simulink model "zoh"  (R2024b)
settings: Solver=VariableStepAuto  StartTime=0.0  StopTime=10.0  RelTol=1e-3
undefined symbols (not defined in the file or in its folder): drv, gbox, mld, mot, PID, rads2rpm, sens, sIn, specs
libraries: simulink_extras x6
settings Model: Creator=Nihal  LastModifiedBy=Nihal

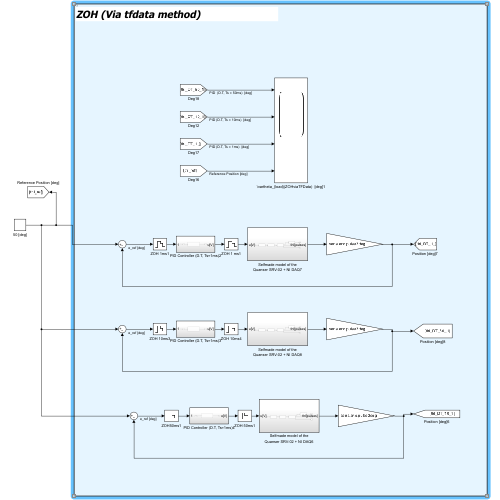
[thumbnail: Simulink's stored preview of the top-level diagram]
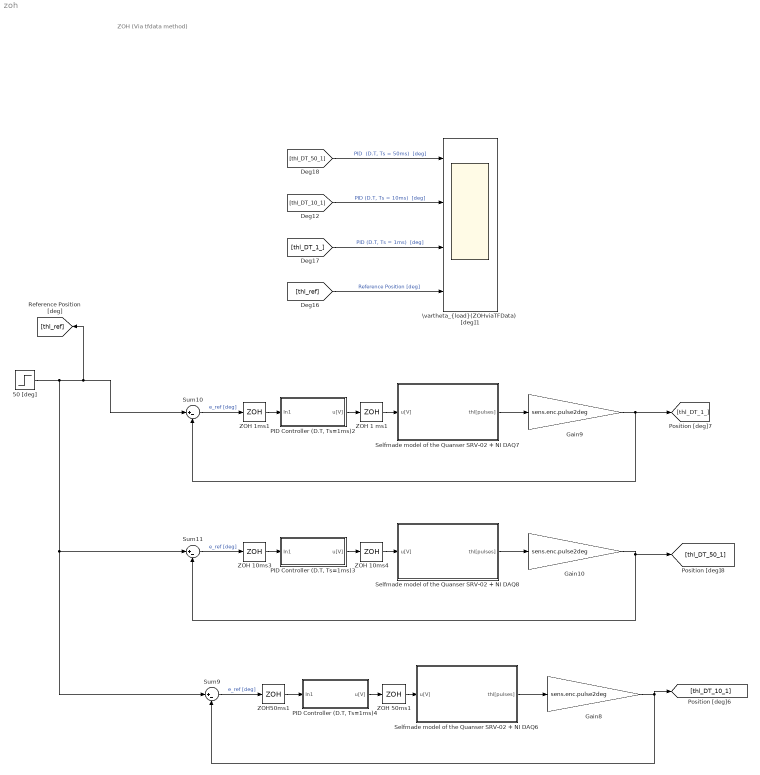
== system zoh ==
  note: ZOH (Via tfdata method)
  50 [deg] : Step  Time=0  After=sIn.position(1)  SampleTime=0
  Gain10 : Gain  Gain=sens.enc.pulse2deg
  Gain8 : Gain  Gain=sens.enc.pulse2deg
  Gain9 : Gain  Gain=sens.enc.pulse2deg
  "PID Controller (D.T, Ts=1ms)2" : Subsystem
  "PID Controller (D.T, Ts=1ms)3" : Subsystem
  "PID Controller (D.T, Ts=1ms)4" : Subsystem
  Selfmade model of the Quanser SRV-02 + NI DAQ6 : Subsystem
  Selfmade model of the Quanser SRV-02 + NI DAQ7 : Subsystem
  Selfmade model of the Quanser SRV-02 + NI DAQ8 : Subsystem
  Sum10 : Sum  Inputs=|+-
  Sum11 : Sum  Inputs=|+-
  Sum9 : Sum  Inputs=|+-
  ZOH 1 ms1 : ZeroOrderHold  SampleTime=specs.Ts(1)
  ZOH 10ms3 : ZeroOrderHold  SampleTime=specs.Ts(2)
  ZOH 10ms4 : ZeroOrderHold  SampleTime=specs.Ts(2)
  ZOH 1ms1 : ZeroOrderHold  SampleTime=specs.Ts(1)
  ZOH 50ms1 : ZeroOrderHold  SampleTime=specs.Ts(3)
  ZOH50ms1 : ZeroOrderHold  SampleTime=specs.Ts(3)
  "\\vartheta_{load}(ZOHviaTFData)  [deg]1" : Scope  NumInputPorts=4
  wires:
  ZOH 50ms1/1 -> Selfmade model of the Quanser SRV-02 + NI DAQ6/1(u[V])
  [thl_DT_50_1] -> "\\vartheta_{load}(ZOHviaTFData)  [deg]1"/1  "PID  (D.T, Ts = 50ms)  [deg]"
  ZOH50ms1/1 -> "PID Controller (D.T, Ts=1ms)4"/1(In1)
  Gain8/1 -> [thl_DT_10_1], Sum9/2
  Sum11/1 -> ZOH 10ms3/1  "e_ref [deg]"
  ZOH 10ms4/1 -> Selfmade model of the Quanser SRV-02 + NI DAQ8/1(u[V])
  "PID Controller (D.T, Ts=1ms)2"/1(u[V]) -> ZOH 1 ms1/1
  Selfmade model of the Quanser SRV-02 + NI DAQ7/1(thl[pulses]) -> Gain9/1
  "PID Controller (D.T, Ts=1ms)4"/1(u[V]) -> ZOH 50ms1/1
  Sum10/1 -> ZOH 1ms1/1  "e_ref [deg]"
  "PID Controller (D.T, Ts=1ms)3"/1(u[V]) -> ZOH 10ms4/1
  ZOH 1ms1/1 -> "PID Controller (D.T, Ts=1ms)2"/1(In1)
  [thl_DT_1_] -> "\\vartheta_{load}(ZOHviaTFData)  [deg]1"/3  "PID (D.T, Ts = 1ms)  [deg]"
  [thl_ref] -> "\\vartheta_{load}(ZOHviaTFData)  [deg]1"/4  "Reference Position [deg]"
  Gain9/1 -> [thl_DT_1_], Sum10/2
  Selfmade model of the Quanser SRV-02 + NI DAQ6/1(thl[pulses]) -> Gain8/1
  ZOH 1 ms1/1 -> Selfmade model of the Quanser SRV-02 + NI DAQ7/1(u[V])
  Sum9/1 -> ZOH50ms1/1  "e_ref [deg]"
  Gain10/1 -> [thl_DT_50_1], Sum11/2
  [thl_DT_10_1] -> "\\vartheta_{load}(ZOHviaTFData)  [deg]1"/2  "PID (D.T, Ts = 10ms)  [deg]"
  ZOH 10ms3/1 -> "PID Controller (D.T, Ts=1ms)3"/1(In1)
  Selfmade model of the Quanser SRV-02 + NI DAQ8/1(thl[pulses]) -> Gain10/1
  50 [deg]/1 -> Sum9/1, Sum11/1, [thl_ref], Sum10/1

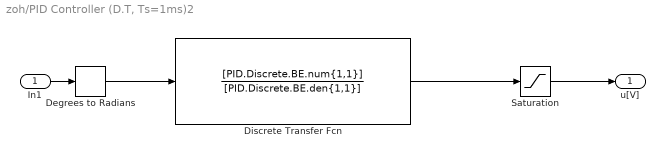
== system zoh/PID Controller (D.T, Ts=1ms)2 ==
  In1 : Inport
  Degrees to Radians : simulink_extras/Transformations/Degrees to Radians
  Discrete Transfer Fcn : DiscreteTransferFcn  Numerator=[PID.Discrete.BE.num{1,1}]  Denominator=[PID.Discrete.BE.den{1,1}]
  Saturation : Saturate  UpperLimit=10  LowerLimit=-10
  u[V] : Outport
  wires:
  In1/1 -> Degrees to Radians/1
  Saturation/1 -> u[V]/1
  Degrees to Radians/1 -> Discrete Transfer Fcn/1
  Discrete Transfer Fcn/1 -> Saturation/1

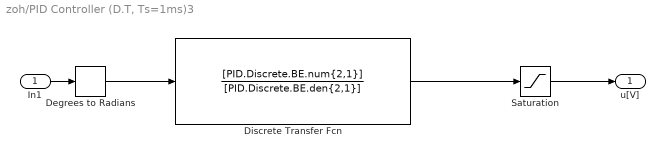
== system zoh/PID Controller (D.T, Ts=1ms)3 ==
  In1 : Inport
  Degrees to Radians : simulink_extras/Transformations/Degrees to Radians
  Discrete Transfer Fcn : DiscreteTransferFcn  Numerator=[PID.Discrete.BE.num{2,1}]  Denominator=[PID.Discrete.BE.den{2,1}]
  Saturation : Saturate  UpperLimit=10  LowerLimit=-10
  u[V] : Outport
  wires:
  In1/1 -> Degrees to Radians/1
  Saturation/1 -> u[V]/1
  Degrees to Radians/1 -> Discrete Transfer Fcn/1
  Discrete Transfer Fcn/1 -> Saturation/1

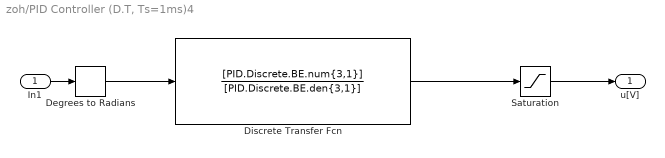
== system zoh/PID Controller (D.T, Ts=1ms)4 ==
  In1 : Inport
  Degrees to Radians : simulink_extras/Transformations/Degrees to Radians
  Discrete Transfer Fcn : DiscreteTransferFcn  Numerator=[PID.Discrete.BE.num{3,1}]  Denominator=[PID.Discrete.BE.den{3,1}]
  Saturation : Saturate  UpperLimit=10  LowerLimit=-10
  u[V] : Outport
  wires:
  In1/1 -> Degrees to Radians/1
  Saturation/1 -> u[V]/1
  Degrees to Radians/1 -> Discrete Transfer Fcn/1
  Discrete Transfer Fcn/1 -> Saturation/1

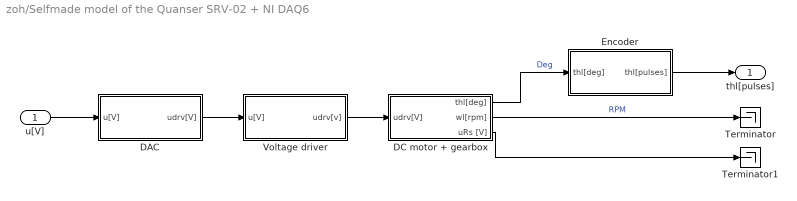
== system zoh/Selfmade model of the Quanser SRV-02 + NI DAQ6 ==
  u[V] : Inport
  DAC : Subsystem
  DC motor + gearbox : Subsystem
  Encoder : Subsystem
  Terminator : Terminator
  Terminator1 : Terminator
  Voltage driver : Subsystem
  thl[pulses] : Outport
  wires:
  DC motor + gearbox/1(thl[deg]) -> Encoder/1(thl[deg])  "Deg"
  u[V]/1 -> DAC/1(u[V])
  DC motor + gearbox/2(wl[rpm]) -> Terminator/1  "RPM"
  DAC/1(udrv[V]) -> Voltage driver/1(u[V])
  Voltage driver/1(udrv[v]) -> DC motor + gearbox/1(udrv[V])
  Encoder/1(thl[pulses]) -> thl[pulses]/1
  DC motor + gearbox/3(uRs [V]) -> Terminator1/1

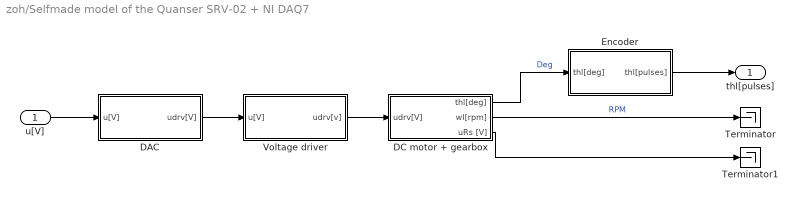
== system zoh/Selfmade model of the Quanser SRV-02 + NI DAQ7 ==
  u[V] : Inport
  DAC : Subsystem
  DC motor + gearbox : Subsystem
  Encoder : Subsystem
  Terminator : Terminator
  Terminator1 : Terminator
  Voltage driver : Subsystem
  thl[pulses] : Outport
  wires:
  DC motor + gearbox/1(thl[deg]) -> Encoder/1(thl[deg])  "Deg"
  u[V]/1 -> DAC/1(u[V])
  DC motor + gearbox/2(wl[rpm]) -> Terminator/1  "RPM"
  DAC/1(udrv[V]) -> Voltage driver/1(u[V])
  Voltage driver/1(udrv[v]) -> DC motor + gearbox/1(udrv[V])
  Encoder/1(thl[pulses]) -> thl[pulses]/1
  DC motor + gearbox/3(uRs [V]) -> Terminator1/1

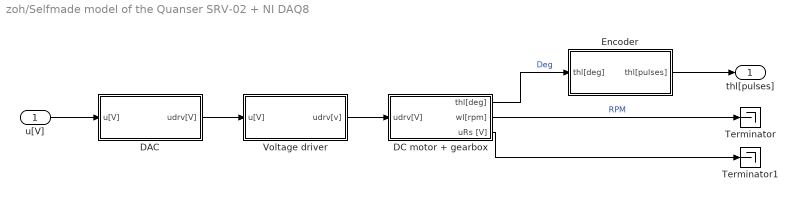
== system zoh/Selfmade model of the Quanser SRV-02 + NI DAQ8 ==
  u[V] : Inport
  DAC : Subsystem
  DC motor + gearbox : Subsystem
  Encoder : Subsystem
  Terminator : Terminator
  Terminator1 : Terminator
  Voltage driver : Subsystem
  thl[pulses] : Outport
  wires:
  DC motor + gearbox/1(thl[deg]) -> Encoder/1(thl[deg])  "Deg"
  u[V]/1 -> DAC/1(u[V])
  DC motor + gearbox/2(wl[rpm]) -> Terminator/1  "RPM"
  DAC/1(udrv[V]) -> Voltage driver/1(u[V])
  Voltage driver/1(udrv[v]) -> DC motor + gearbox/1(udrv[V])
  Encoder/1(thl[pulses]) -> thl[pulses]/1
  DC motor + gearbox/3(uRs [V]) -> Terminator1/1

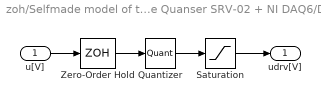
== system zoh/Selfmade model of the Quanser SRV-02 + NI DAQ6/DAC ==
  u[V] : Inport
  Quantizer : Quantizer  QuantizationInterval=daq.dac.q
  Saturation : Saturate  UpperLimit=10  LowerLimit=-10
  Zero-Order Hold : ZeroOrderHold  SampleTime=1e-3
  udrv[V] : Outport
  wires:
  Zero-Order Hold/1 -> Quantizer/1
  u[V]/1 -> Zero-Order Hold/1
  Quantizer/1 -> Saturation/1
  Saturation/1 -> udrv[V]/1

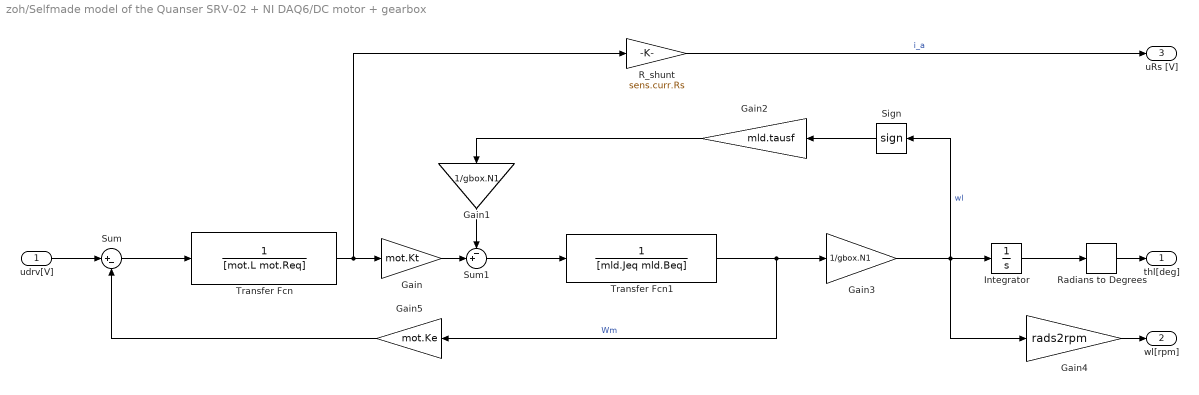
== system zoh/Selfmade model of the Quanser SRV-02 + NI DAQ6/DC motor + gearbox ==
  udrv[V] : Inport
  Gain : Gain  Gain=mot.Kt
  Gain1 : Gain  Gain=1/gbox.N1
  Gain2 : Gain  Gain=mld.tausf
  Gain3 : Gain  Gain=1/gbox.N1
  Gain4 : Gain  Gain=rads2rpm
  Gain5 : Gain  Gain=mot.Ke
  Integrator : Integrator
  R_shunt : Gain  Gain=sens.curr.Rs
  Radians to Degrees : simulink_extras/Transformations/Radians to Degrees
  Sign : Signum  ZeroCross=off
  Sum : Sum  Inputs=|+-
  Sum1 : Sum  Inputs=-+|
  Transfer Fcn : TransferFcn  Denominator=[mot.L mot.Req]
  Transfer Fcn1 : TransferFcn  Denominator=[mld.Jeq mld.Beq]
  thl[deg] : Outport
  wl[rpm] : Outport  Port=2
  uRs [V] : Outport  Port=3
  wires:
  udrv[V]/1 -> Sum/1
  Sum/1 -> Transfer Fcn/1
  Transfer Fcn/1 -> R_shunt/1, Gain/1
  Gain1/1 -> Sum1/1
  Gain2/1 -> Gain1/1
  Sign/1 -> Gain2/1
  Transfer Fcn1/1 -> Gain5/1, Gain3/1  "Wm"
  Gain3/1 -> Gain4/1, Sign/1, Integrator/1  "wl"
  Integrator/1 -> Radians to Degrees/1
  Radians to Degrees/1 -> thl[deg]/1
  Gain4/1 -> wl[rpm]/1
  Sum1/1 -> Transfer Fcn1/1
  Gain/1 -> Sum1/2
  Gain5/1 -> Sum/2
  R_shunt/1 -> uRs [V]/1  "i_a"

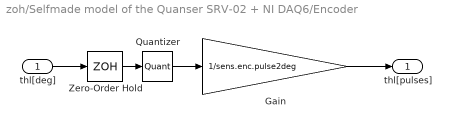
== system zoh/Selfmade model of the Quanser SRV-02 + NI DAQ6/Encoder ==
  thl[deg] : Inport
  Gain : Gain  Gain=1/sens.enc.pulse2deg
  Quantizer : Quantizer  QuantizationInterval=sens.enc.pulse2deg
  Zero-Order Hold : ZeroOrderHold  SampleTime=1e-3
  thl[pulses] : Outport
  wires:
  thl[deg]/1 -> Zero-Order Hold/1
  Gain/1 -> thl[pulses]/1
  Quantizer/1 -> Gain/1
  Zero-Order Hold/1 -> Quantizer/1

== system zoh/Selfmade model of the Quanser SRV-02 + NI DAQ6/Voltage driver ==
  u[V] : Inport
  Saturation : Saturate  UpperLimit=12  LowerLimit=-12
  Transfer Fcn : TransferFcn  Numerator=[drv.dcgain]  Denominator=[drv.Tc 1]
  udrv[v] : Outport
  wires:
  u[V]/1 -> Transfer Fcn/1
  Transfer Fcn/1 -> Saturation/1
  Saturation/1 -> udrv[v]/1

== system zoh/Selfmade model of the Quanser SRV-02 + NI DAQ7/DAC ==
  u[V] : Inport
  Quantizer : Quantizer  QuantizationInterval=daq.dac.q
  Saturation : Saturate  UpperLimit=10  LowerLimit=-10
  Zero-Order Hold : ZeroOrderHold  SampleTime=1e-3
  udrv[V] : Outport
  wires:
  Zero-Order Hold/1 -> Quantizer/1
  u[V]/1 -> Zero-Order Hold/1
  Quantizer/1 -> Saturation/1
  Saturation/1 -> udrv[V]/1

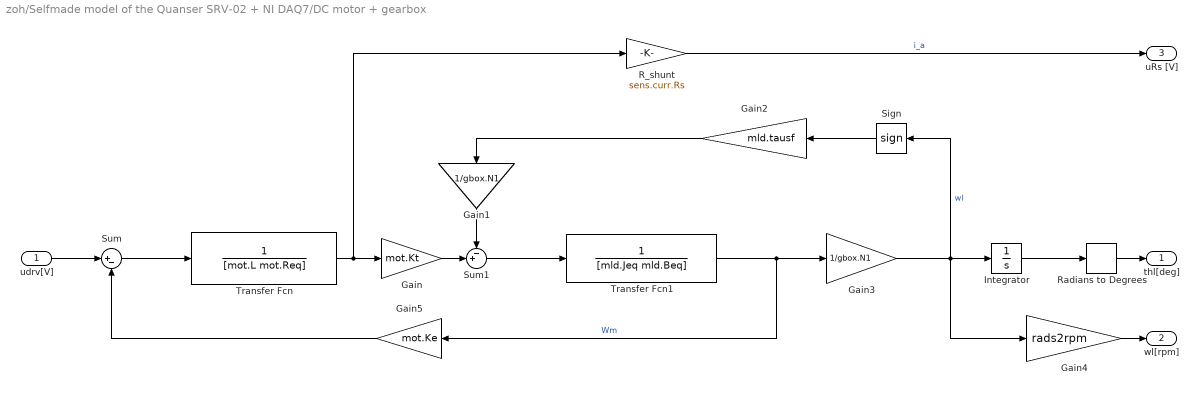
== system zoh/Selfmade model of the Quanser SRV-02 + NI DAQ7/DC motor + gearbox ==
  udrv[V] : Inport
  Gain : Gain  Gain=mot.Kt
  Gain1 : Gain  Gain=1/gbox.N1
  Gain2 : Gain  Gain=mld.tausf
  Gain3 : Gain  Gain=1/gbox.N1
  Gain4 : Gain  Gain=rads2rpm
  Gain5 : Gain  Gain=mot.Ke
  Integrator : Integrator
  R_shunt : Gain  Gain=sens.curr.Rs
  Radians to Degrees : simulink_extras/Transformations/Radians to Degrees
  Sign : Signum  ZeroCross=off
  Sum : Sum  Inputs=|+-
  Sum1 : Sum  Inputs=-+|
  Transfer Fcn : TransferFcn  Denominator=[mot.L mot.Req]
  Transfer Fcn1 : TransferFcn  Denominator=[mld.Jeq mld.Beq]
  thl[deg] : Outport
  wl[rpm] : Outport  Port=2
  uRs [V] : Outport  Port=3
  wires:
  udrv[V]/1 -> Sum/1
  Sum/1 -> Transfer Fcn/1
  Transfer Fcn/1 -> R_shunt/1, Gain/1
  Gain1/1 -> Sum1/1
  Gain2/1 -> Gain1/1
  Sign/1 -> Gain2/1
  Transfer Fcn1/1 -> Gain5/1, Gain3/1  "Wm"
  Gain3/1 -> Gain4/1, Sign/1, Integrator/1  "wl"
  Integrator/1 -> Radians to Degrees/1
  Radians to Degrees/1 -> thl[deg]/1
  Gain4/1 -> wl[rpm]/1
  Sum1/1 -> Transfer Fcn1/1
  Gain/1 -> Sum1/2
  Gain5/1 -> Sum/2
  R_shunt/1 -> uRs [V]/1  "i_a"

== system zoh/Selfmade model of the Quanser SRV-02 + NI DAQ7/Encoder ==
  thl[deg] : Inport
  Gain : Gain  Gain=1/sens.enc.pulse2deg
  Quantizer : Quantizer  QuantizationInterval=sens.enc.pulse2deg
  Zero-Order Hold : ZeroOrderHold  SampleTime=1e-3
  thl[pulses] : Outport
  wires:
  thl[deg]/1 -> Zero-Order Hold/1
  Gain/1 -> thl[pulses]/1
  Quantizer/1 -> Gain/1
  Zero-Order Hold/1 -> Quantizer/1

== system zoh/Selfmade model of the Quanser SRV-02 + NI DAQ7/Voltage driver ==
  u[V] : Inport
  Saturation : Saturate  UpperLimit=12  LowerLimit=-12
  Transfer Fcn : TransferFcn  Numerator=[drv.dcgain]  Denominator=[drv.Tc 1]
  udrv[v] : Outport
  wires:
  u[V]/1 -> Transfer Fcn/1
  Transfer Fcn/1 -> Saturation/1
  Saturation/1 -> udrv[v]/1

== system zoh/Selfmade model of the Quanser SRV-02 + NI DAQ8/DAC ==
  u[V] : Inport
  Quantizer : Quantizer  QuantizationInterval=daq.dac.q
  Saturation : Saturate  UpperLimit=10  LowerLimit=-10
  Zero-Order Hold : ZeroOrderHold  SampleTime=1e-3
  udrv[V] : Outport
  wires:
  Zero-Order Hold/1 -> Quantizer/1
  u[V]/1 -> Zero-Order Hold/1
  Quantizer/1 -> Saturation/1
  Saturation/1 -> udrv[V]/1

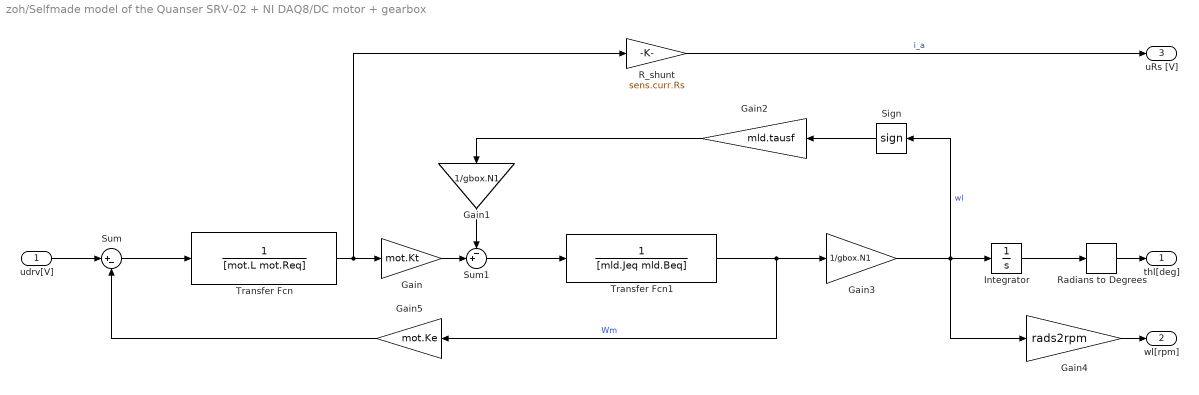
== system zoh/Selfmade model of the Quanser SRV-02 + NI DAQ8/DC motor + gearbox ==
  udrv[V] : Inport
  Gain : Gain  Gain=mot.Kt
  Gain1 : Gain  Gain=1/gbox.N1
  Gain2 : Gain  Gain=mld.tausf
  Gain3 : Gain  Gain=1/gbox.N1
  Gain4 : Gain  Gain=rads2rpm
  Gain5 : Gain  Gain=mot.Ke
  Integrator : Integrator
  R_shunt : Gain  Gain=sens.curr.Rs
  Radians to Degrees : simulink_extras/Transformations/Radians to Degrees
  Sign : Signum  ZeroCross=off
  Sum : Sum  Inputs=|+-
  Sum1 : Sum  Inputs=-+|
  Transfer Fcn : TransferFcn  Denominator=[mot.L mot.Req]
  Transfer Fcn1 : TransferFcn  Denominator=[mld.Jeq mld.Beq]
  thl[deg] : Outport
  wl[rpm] : Outport  Port=2
  uRs [V] : Outport  Port=3
  wires:
  udrv[V]/1 -> Sum/1
  Sum/1 -> Transfer Fcn/1
  Transfer Fcn/1 -> R_shunt/1, Gain/1
  Gain1/1 -> Sum1/1
  Gain2/1 -> Gain1/1
  Sign/1 -> Gain2/1
  Transfer Fcn1/1 -> Gain5/1, Gain3/1  "Wm"
  Gain3/1 -> Gain4/1, Sign/1, Integrator/1  "wl"
  Integrator/1 -> Radians to Degrees/1
  Radians to Degrees/1 -> thl[deg]/1
  Gain4/1 -> wl[rpm]/1
  Sum1/1 -> Transfer Fcn1/1
  Gain/1 -> Sum1/2
  Gain5/1 -> Sum/2
  R_shunt/1 -> uRs [V]/1  "i_a"

== system zoh/Selfmade model of the Quanser SRV-02 + NI DAQ8/Encoder ==
  thl[deg] : Inport
  Gain : Gain  Gain=1/sens.enc.pulse2deg
  Quantizer : Quantizer  QuantizationInterval=sens.enc.pulse2deg
  Zero-Order Hold : ZeroOrderHold  SampleTime=1e-3
  thl[pulses] : Outport
  wires:
  thl[deg]/1 -> Zero-Order Hold/1
  Gain/1 -> thl[pulses]/1
  Quantizer/1 -> Gain/1
  Zero-Order Hold/1 -> Quantizer/1

== system zoh/Selfmade model of the Quanser SRV-02 + NI DAQ8/Voltage driver ==
  u[V] : Inport
  Saturation : Saturate  UpperLimit=12  LowerLimit=-12
  Transfer Fcn : TransferFcn  Numerator=[drv.dcgain]  Denominator=[drv.Tc 1]
  udrv[v] : Outport
  wires:
  u[V]/1 -> Transfer Fcn/1
  Transfer Fcn/1 -> Saturation/1
  Saturation/1 -> udrv[v]/1
